simulink model "PID_conlac"  (R2019a)
settings: Solver=ode5  StartTime=0.0  StopTime=20  FixedStep=0.01  RelTol=1e-3
undefined symbols (not defined in the file): sigbuilder_block
libraries: fuzblock x1
settings Model: Creator=forev  LastModifiedBy=forev

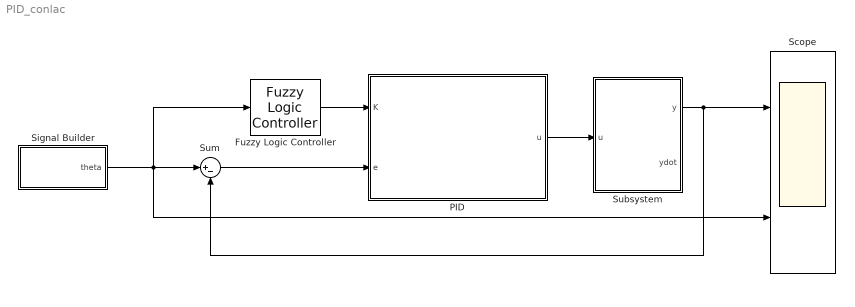
== system PID_conlac ==
  Fuzzy Logic Controller : fuzblock/Fuzzy Logic  Controller  FIS='PID_conlac.fis'  OutputSampleNumber=101  DataType=double  FuzzifiedInputs=off  RuleFiringStrengths=off  RuleOutputs=off  AggregatedOutputs=off  SimulateUsing=Interpreted execution  OutOfRangeInputValueMessage=warning  NoRuleFiredMessage=warning  EmptyOutputFuzzySetMessage=warning
  PID : Subsystem
  Scope : Scope  NumInputPorts=2
  Signal Builder : Subsystem  Tag=STV Subsys  LoadFcn=sigbuilder_block('load');  StartFcn=sigbuilder_block('start');  StopFcn=sigbuilder_block('stop');  ClipboardFcn=sigbuilder_block('clipboard');  mask(Sigbuilder block){tuvar=[0:10]}
      mask help: Simulink:masks:SigbuilderBlock_MD
      mask init:
      | if ~strcmp(get_param(bdroot(gcbh),'SimulationStatus'),'stopped') tuvar = sigbuilder_block('maskInit'); end
      settings: CopyFcn=sigbuilder_block('copy');  DeleteFcn=sigbuilder_block('delete');  ModelCloseFcn=sigbuilder_block('modelClose');  PreSaveFcn=sigbuilder_block('preSave');  PauseFcn=sigbuilder_block('pause');  ContinueFcn=sigbuilder_block('continue');  NameChangeFcn=sigbuilder_block('namechange');  OpenFcn=sigbuilder_block('open',[5.4 30 1141.2 522.6 ]);  CloseFcn=sigbuilder_block('close');
      mask Display: plot(0, 0, 100, 100,[2, 2, 32, 32, 2], [68, 8, 8, 68, 68],[32, 2], [38, 38], [32, 19, 2],[53, 60, 44], [32, 17, 17, 2],[16, 16, 31, 31]);txt = getActiveGroup(gcbh);text(2, 100, txt,'verticalAlignment', 'top');
  Subsystem : Subsystem  mask{m=0.5, k=0.1, l=0.6, g=9.81, y0=0, ydot0=0, b=0.1, theta_dot0=0}
      mask prompts: m "trọng lượng con lac"; k "trong lượng con lắc"; l "chiều dài con lắc"; g "gia tốc trọng trường"; y0 "vị trí ban đầu"; ydot0 "vận tốc ban đầu"; b "he so ma sat"; theta_dot0 "vận tốc góc ban đầu"
  Sum : Sum  Inputs=|+-
  wires:
  Signal Builder/1(theta) -> Scope/2, Fuzzy Logic Controller/1, Sum/1
  Sum/1 -> PID/2(e)
  PID/1(u) -> Subsystem/1(u)
  Subsystem/1(y) -> Sum/2, Scope/1
  Fuzzy Logic Controller/1 -> PID/1(K)

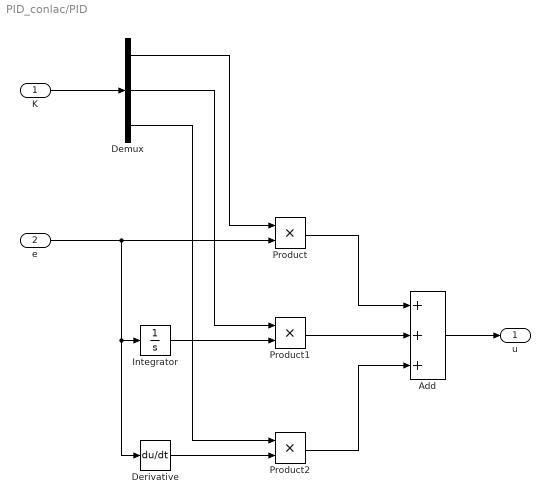
== system PID_conlac/PID ==
  K : Inport
  e : Inport  Port=2
  Add : Sum  Inputs=+++
  Demux : Demux  Outputs=3
  Derivative : Derivative
  Integrator : Integrator
  Product : Product
  Product1 : Product
  Product2 : Product
  u : Outport
  wires:
  K/1 -> Demux/1
  Demux/1 -> Product/1
  e/1 -> Derivative/1, Integrator/1, Product/2
  Integrator/1 -> Product1/2
  Demux/2 -> Product1/1
  Derivative/1 -> Product2/2
  Demux/3 -> Product2/1
  Add/1 -> u/1
  Product/1 -> Add/1
  Product1/1 -> Add/2
  Product2/1 -> Add/3

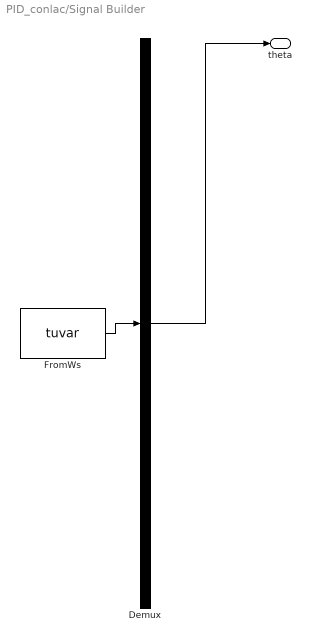
== system PID_conlac/Signal Builder ==
  Demux : Demux  Tag=STV Demux  Outputs=1
  FromWs : FromWorkspace  Tag=STV FromWs  VariableName=tuvar  SampleTime=0
      SigBuilderData=|
      | common.afterFinalStr = 'Extrapolate'
      | common.sampleTime = 0
      | dataSet.timeRange = [0 20]
      | dataSet.name = 'Group 1'
      | sbobj.Groups.Name = 'Group 1'
      | sbobj.Groups.Signals.Name = 'theta'
      | sbobj.Groups.Signals.XData = [0 0.96 0.96 20]
      | sbobj.Groups.Signals.YData = [0 0 2.09333333333 2.09333333333]
      | sbobj.Groups.TimeRange = [0 20]
  theta : Outport  Tag=STV Outport
  wires:
  Demux/1 -> theta/1
  FromWs/1 -> Demux/1

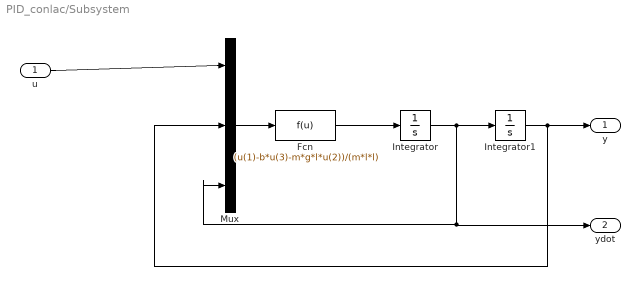
== system PID_conlac/Subsystem ==
  u : Inport
  Fcn : Fcn  Expr=(u(1)-b*u(3)-m*g*l*u(2))/(m*l*l)
  Integrator : Integrator  InitialCondition=ydot0
  Integrator1 : Integrator  InitialCondition=y0
  Mux : Mux  Inputs=3
  y : Outport
  ydot : Outport  Port=2
  wires:
  Integrator/1 -> ydot/1, Mux/3, Integrator1/1
  Mux/1 -> Fcn/1
  u/1 -> Mux/1
  Integrator1/1 -> Mux/2, y/1
  Fcn/1 -> Integrator/1
